simulink subsystem "Scenario_Command"  (R2025a)
settings: Solver=VariableStepAuto  StartTime=0.0  StopTime=10.0  RelTol=1e-3
undefined symbols (not defined in the file): config
settings Model: Creator=Jackt  LastModifiedBy=Jackt

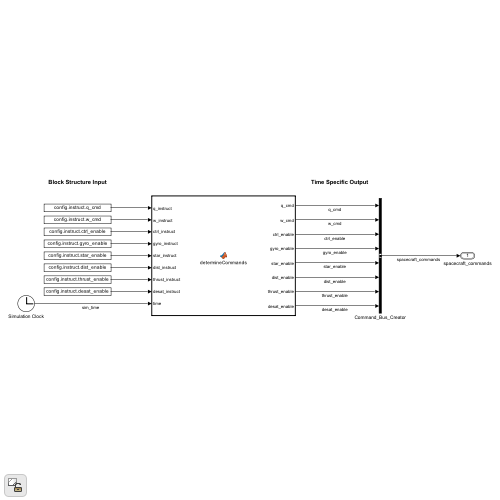
[thumbnail: Simulink's stored preview of the top-level diagram]
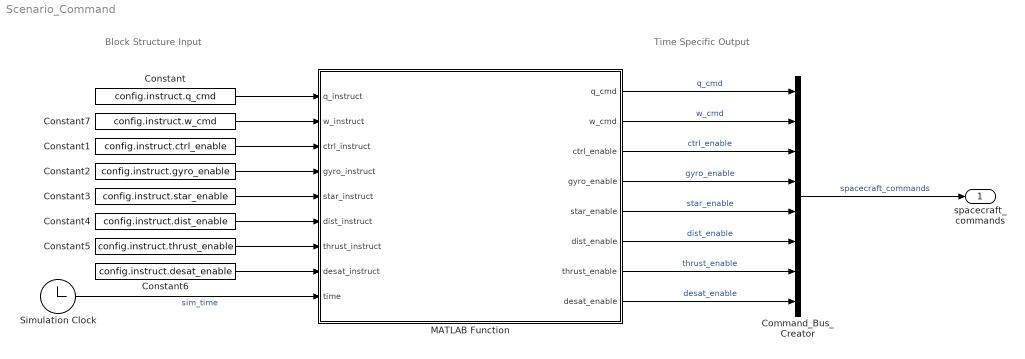
== system Scenario_Command ==
  note: Block Structure Input
  note: Time Specific Output
  Command_Bus_Creator : BusCreator  Inputs=8  OutDataTypeStr=Bus: commandBus
  Constant : Constant  Value=config.instruct.q_cmd  VectorParams1D=off  OutDataTypeStr=double
  Constant1 : Constant  Value=config.instruct.ctrl_enable  VectorParams1D=off  OutDataTypeStr=double
  Constant2 : Constant  Value=config.instruct.gyro_enable  VectorParams1D=off  OutDataTypeStr=double
  Constant3 : Constant  Value=config.instruct.star_enable  VectorParams1D=off  OutDataTypeStr=double
  Constant4 : Constant  Value=config.instruct.dist_enable  VectorParams1D=off  OutDataTypeStr=double
  Constant5 : Constant  Value=config.instruct.thrust_enable  VectorParams1D=off  OutDataTypeStr=double
  Constant6 : Constant  Value=config.instruct.desat_enable  VectorParams1D=off  OutDataTypeStr=double
  Constant7 : Constant  Value=config.instruct.w_cmd  VectorParams1D=off  OutDataTypeStr=double
  MATLAB Function : MATLAB Function  TreatAsAtomicUnit=on
  Simulation Clock : Clock
  spacecraft_commands : Outport  OutDataTypeStr=Bus: commandBus
  wires:
  Simulation Clock/1 -> MATLAB Function/9(time)  "sim_time"
  MATLAB Function/1(q_cmd) -> Command_Bus_Creator/1  "q_cmd"
  MATLAB Function/2(w_cmd) -> Command_Bus_Creator/2  "w_cmd"
  MATLAB Function/3(ctrl_enable) -> Command_Bus_Creator/3  "ctrl_enable"
  MATLAB Function/4(gyro_enable) -> Command_Bus_Creator/4  "gyro_enable"
  MATLAB Function/5(star_enable) -> Command_Bus_Creator/5  "star_enable"
  MATLAB Function/6(dist_enable) -> Command_Bus_Creator/6  "dist_enable"
  MATLAB Function/7(thrust_enable) -> Command_Bus_Creator/7  "thrust_enable"
  MATLAB Function/8(desat_enable) -> Command_Bus_Creator/8  "desat_enable"
  Command_Bus_Creator/1 -> spacecraft_commands/1  "spacecraft_commands"
  Constant/1 -> MATLAB Function/1(q_instruct)
  Constant1/1 -> MATLAB Function/3(ctrl_instruct)
  Constant2/1 -> MATLAB Function/4(gyro_instruct)
  Constant6/1 -> MATLAB Function/8(desat_instruct)
  Constant5/1 -> MATLAB Function/7(thrust_instruct)
  Constant4/1 -> MATLAB Function/6(dist_instruct)
  Constant3/1 -> MATLAB Function/5(star_instruct)
  Constant7/1 -> MATLAB Function/2(w_instruct)

== matlab function Scenario_Command/MATLAB Function ==
  data: q_instruct input; w_instruct input; ctrl_instruct input; gyro_instruct input; star_instruct input; dist_instruct input; thrust_instruct input; desat_instruct input; q_cmd output double size=[4,1]; w_cmd output double size=[3, 1]; ctrl_enable output double size=1; gyro_enable output double size=1; star_enable output double size=1; dist_enable output double size=1; thrust_enable output double size=1; desat_enable output double size=1; time input
function [q_cmd, w_cmd, ctrl_enable, gyro_enable, star_enable, dist_enable, thrust_enable, desat_enable] = determineCommands(q_instruct, w_instruct, ctrl_instruct, gyro_instruct, star_instruct, dist_instruct, thrust_instruct, desat_instruct, time)
%DETERMINECOMMANDS Function processes run-time command structures to
%determine what commands should be sent to the spacecraft for any given
%time

% Pre-allocate output variable sizes
q_cmd = zeros(4,1);
w_cmd = zeros(3,1);

ctrl_enable   = 0;
gyro_enable   = 0;
star_enable   = 0;
dist_enable   = 0;
thrust_enable = 0;
desat_enable  = 0;

%% Quaternion Position Instructions
timeCol = q_instruct(:, 1); %[seconds]
index = find(timeCol <= time, 1, 'last');
if(isempty(index)); index = 1; end
q_cmd(1:4) = q_instruct(index, 2:5);

%% Angular Rate Instructions
timeCol = w_instruct(:, 1); %[seconds]
index = find(timeCol <= time, 1, 'last');
if(isempty(index)); index = 1; end
w_cmd = w_instruct(index, 2:end);

%% Controller Enabled Instructions
timeCol = ctrl_instruct(:, 1); %[seconds]
index = find(timeCol <= time, 1, 'last');
if(isempty(index)); index = 1; end
ctrl_enable = ctrl_instruct(index, 2:end);

%% Gyroscope Enabled Instructions
timeCol = gyro_instruct(:, 1); %[seconds]
index = find(timeCol <= time, 1, 'last');
if(isempty(index)); index = 1; end
gyro_enable = gyro_instruct(index, 2:end);

%% Star Tracker Enabled Instructions
timeCol = star_instruct(:, 1); %[seconds]
index = find(timeCol <= time, 1, 'last');
if(isempty(index)); index = 1; end
star_enable = star_instruct(index, 2:end);

%% Disturbances Enabled Instructions
timeCol = dist_instruct(:, 1); %[seconds]
index = find(timeCol <= time, 1, 'last');
if(isempty(index)); index = 1; end
dist_enable = dist_instruct(index, 2:end);

%% Thruster Enabled Instructions
timeCol = thrust_instruct(:, 1); %[seconds]
index = find(timeCol <= time, 1, 'last');
if(isempty(index)); index = 1; end
thrust_enable = thrust_instruct(index, 2:end);

%% Desaturation Enabled Instructions
timeCol = desat_instruct(:, 1); %[seconds]
index = find(timeCol <= time, 1, 'last');
if(isempty(index)); index = 1; end
desat_enable = desat_instruct(index, 2:end);

%% Assign Output Variable Sizes for Simulink
q_cmd = reshape(q_cmd, [4 1]);
w_cmd = reshape(w_cmd, [3 1]);
ctrl_enable  = double(ctrl_enable(1));
gyro_enable  = double(gyro_enable(1));
star_enable  = double(star_enable(1));
dist_enable  = double(dist_enable(1));
thrust_enable= double(thrust_enable(1));
desat_enable = double(desat_enable(1));
end
